simulink model "Drone_Flight_Model_StandAlone_KF_Steady"  (R2016b)
settings: Solver=FixedStepDiscrete  StartTime=0.0  StopTime=20  FixedStep=1/400  RelTol=1e-3  EnableMultiTasking=on
model workspace: external: MAT-File C:\Users\Patrick\Documents\TU\Integration project\AR_Drone_Models\Flight_Models\PD\parameters.mat (data not in the file)
undefined symbols (not defined in the file): accelerometerXyzGains, accelerometerXyzOffsets, Ak, Bk, botCamData, Ck, D_height, D_pitch, D_roll, D_yaw, DiscIntNeverNeededParam, Dk, Drone_StateModeType, dronePowerScaling, g, gyroXyzOffsets, I_height, M, magnetoXyzOffsets, Mass, P_height, P_pitch, P_roll, P_yaw, propDistance, yawTorqueC
libraries: simulink x17, dspstat3 x3, AR_Drone_Sensors x3, AR_Drone_Actuators x3, dspnetwork x2, visionanalysis x2, vrlib x2, AR_Drone_Video x1, AR_Drone_Positioning x1
(part 1 of 2)
settings Model: DataDictionary=ArDroneDataDictionary.sldd  ExtModeTrigDuration=48000  ExtModeLogAll=off  Creator=nraman  LastModifiedBy=s136161
settings ConfigSet: Description=This configuration set can be used to generate code that runs on the Parrot AR Drone 2.0 in Normal mode.
settings SolverCC: PositivePriorityOrder=on
settings DataIOCC: LimitDataPoints=on  SaveFormat=Array
settings OptimizationCC: DefaultParameterBehavior=Inlined  InlineInvariantSignals=on  LifeSpan=1  MaxStackSize=64
settings DebuggingCC: UnderspecifiedInitializationDetection=Classic  MergeDetectMultiDrivingBlocksExec=none  SFUnexpectedBacktrackingDiag=warning  SFNoUnconditionalDefaultTransitionDiag=warning
settings HardwareCC: ProdBitPerPointer=32  ProdBitPerSizeT=32  ProdBitPerPtrDiffT=32  ProdLargestAtomicInteger=Long  ProdLargestAtomicFloat=Double  ProdIntDivRoundTo=Undefined  ProdWordSize=32  ProdHWDeviceType=ARM Compatible->ARM Cortex
settings ModelReferenceCC: PropagateSignalLabelsOutOfModel=off
settings SFSimCC: SimUserSources=ArClock.c
settings SFSimCC: SimCustomHeaderCode=|
  | #include "IMU_Navdata.h"
  | #include "ArClock.h"
settings RTWCC: SystemTargetFile=ert.tlc  HardwareBoard=AR Drone 2 - Thread Timer Scheduler  TLCOptions=-aInlineSetEventsForThisBaseRateFcn=TLC_FALSE -aSuppressMultiTaskScheduler=TLC_FALSE -aRateBasedStepFcn=0  TemplateMakefile=ert_default_tmf  Description=Embedded Coder  RTWUseSimCustomCode=on  CustomSource=ArClock.c  Toolchain=Code Sourcery  BuildConfiguration=Faster Runs
settings RTWCC: CustomHeaderCode=|
  | #include "IMU_Navdata.h"
  | #include "ArClock.h"
settings CodeAppCC: IgnoreCustomStorageClasses=off
settings ERTTargetCC: SupportComplex=off  SupportVariableSizeSignals=on  ExtModeMexArgs='192.168.1.1' 1 17725  SuppressUnreachableDefaultCases=off
settings ConfigComp: CovMetricSettings=dw  CovHtmlReporting=on  CovSaveCumulativeToWorkspaceVar=on  CovSaveSingleToWorkspaceVar=on  CovExternalEMLEnable=off

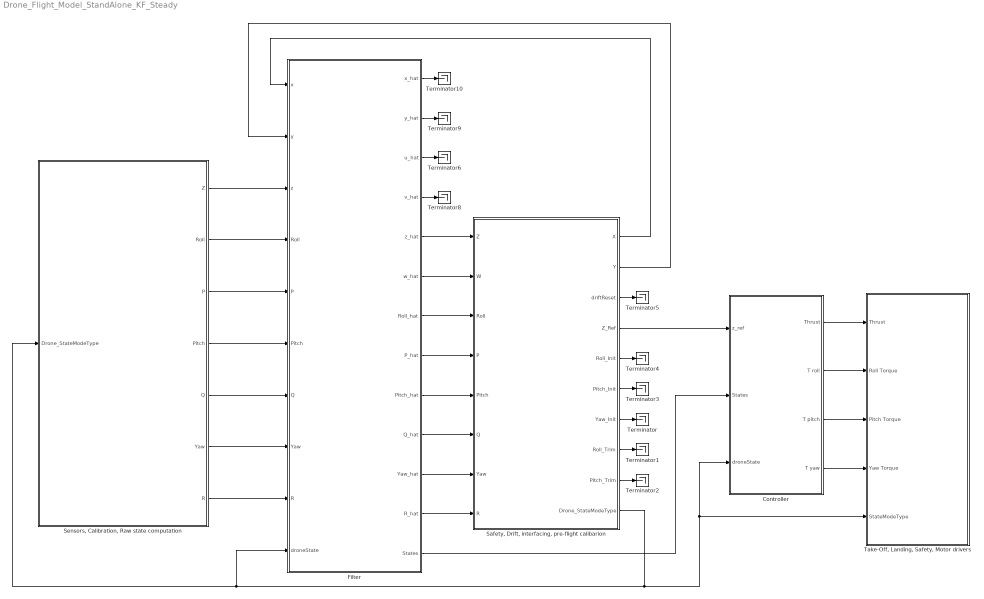
== system Drone_Flight_Model_StandAlone_KF_Steady ==
  Controller : Subsystem
  Filter : Subsystem
  "Safety, Drift, interfacing, pre-flight calibarion" : Subsystem
      settings: OpenFcn=msgbox('Please do not alter the functionality in the pre-made blocks.','Warning');
  "Sensors, Calibration, Raw state computation" : Subsystem
      settings: OpenFcn=msgbox('Please do not alter the functionality in the pre-made blocks.','Warning');
  "Take-Off, Landing, Safety, Motor drivers" : Subsystem
      settings: OpenFcn=msgbox('Please do not alter the functionality in the pre-made blocks.','Warning');
  Terminator{,1..6,8..10} (10 alike) : Terminator
  wires:
  "Safety, Drift, interfacing, pre-flight calibarion"/10(Drone_StateModeType) -> Filter/10(droneState), "Sensors, Calibration, Raw state computation"/1(Drone_StateModeType), Controller/3(droneState), "Take-Off, Landing, Safety, Motor drivers"/5(StateModeType)
  "Sensors, Calibration, Raw state computation"/1(Z) -> Filter/3(z)
  Filter/12(R_hat) -> "Safety, Drift, interfacing, pre-flight calibarion"/8(R)
  Filter/11(Yaw_hat) -> "Safety, Drift, interfacing, pre-flight calibarion"/7(Yaw)
  Filter/10(Q_hat) -> "Safety, Drift, interfacing, pre-flight calibarion"/6(Q)
  Filter/9(Pitch_hat) -> "Safety, Drift, interfacing, pre-flight calibarion"/5(Pitch)
  Filter/8(P_hat) -> "Safety, Drift, interfacing, pre-flight calibarion"/4(P)
  Filter/7(Roll_hat) -> "Safety, Drift, interfacing, pre-flight calibarion"/3(Roll)
  "Sensors, Calibration, Raw state computation"/2(Roll) -> Filter/4(Roll)
  "Sensors, Calibration, Raw state computation"/4(Pitch) -> Filter/6(Pitch)
  "Sensors, Calibration, Raw state computation"/3(P) -> Filter/5(P)
  "Sensors, Calibration, Raw state computation"/5(Q) -> Filter/7(Q)
  "Sensors, Calibration, Raw state computation"/6(Yaw) -> Filter/8(Yaw)
  "Sensors, Calibration, Raw state computation"/7(R) -> Filter/9(R)
  Filter/5(z_hat) -> "Safety, Drift, interfacing, pre-flight calibarion"/1(Z)
  "Safety, Drift, interfacing, pre-flight calibarion"/1(X) -> Filter/1(x)
  "Safety, Drift, interfacing, pre-flight calibarion"/2(Y) -> Filter/2(y)
  "Safety, Drift, interfacing, pre-flight calibarion"/9(Pitch_Trim) -> Terminator2/1
  "Safety, Drift, interfacing, pre-flight calibarion"/8(Roll_Trim) -> Terminator1/1
  "Safety, Drift, interfacing, pre-flight calibarion"/7(Yaw_Init) -> Terminator/1
  "Safety, Drift, interfacing, pre-flight calibarion"/6(Pitch_Init) -> Terminator3/1
  "Safety, Drift, interfacing, pre-flight calibarion"/5(Roll_Init) -> Terminator4/1
  "Safety, Drift, interfacing, pre-flight calibarion"/3(driftReset) -> Terminator5/1
  Filter/6(w_hat) -> "Safety, Drift, interfacing, pre-flight calibarion"/2(W)
  "Safety, Drift, interfacing, pre-flight calibarion"/4(Z_Ref) -> Controller/1(z_ref)
  Filter/13(States) -> Controller/2(States)
  Controller/1(Thrust) -> "Take-Off, Landing, Safety, Motor drivers"/1(Thrust)
  Controller/2(T roll) -> "Take-Off, Landing, Safety, Motor drivers"/2(Roll Torque)
  Controller/3(T pitch) -> "Take-Off, Landing, Safety, Motor drivers"/3(Pitch Torque)
  Controller/4(T yaw) -> "Take-Off, Landing, Safety, Motor drivers"/4(Yaw Torque)
  Filter/1(x_hat) -> Terminator10/1
  Filter/2(y_hat) -> Terminator9/1
  Filter/3(u_hat) -> Terminator6/1
  Filter/4(v_hat) -> Terminator8/1

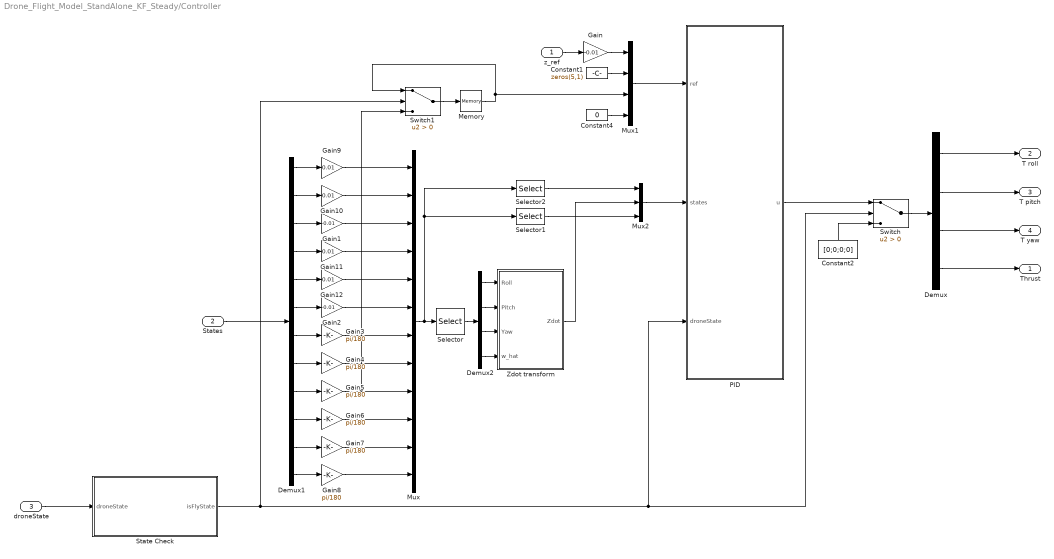
== system Drone_Flight_Model_StandAlone_KF_Steady/Controller ==
  z_ref : Inport
  States : Inport  Port=2
  droneState : Inport  Port=3
  Constant1 : Constant  Value=zeros(5,1)
  Constant2 : Constant  Value=[0;0;0;0]
  Constant4 : Constant  Value=0
  Demux : Demux
  Demux1 : Demux  Outputs=12
  Demux2 : Demux
  Gain : Gain  Gain=-0.01
  Gain1 : Gain  Gain=-0.01
  Gain{9..12} (4 alike) : Gain  Gain=0.01
  Gain2 : Gain  Gain=-0.01
  Gain{3..8} (6 alike) : Gain  Gain=pi/180
  Memory : Memory
  Mux : Mux  Inputs=12
  Mux1 : Mux
  Mux2 : Mux  Inputs=3
  PID : Subsystem
  Selector : Selector  InputPortWidth=12  IndexOptions=Index vector (dialog)  Indices=[7 8 9 6]  OutputSizes=1
  Selector1 : Selector  InputPortWidth=12  IndexOptions=Index vector (dialog)  Indices=[7 10 8 11 9 12]  OutputSizes=1
  Selector2 : Selector  InputPortWidth=12  IndexOptions=Index vector (dialog)  Indices=[3]  OutputSizes=1
  State Check : Subsystem
  Switch : Switch  Criteria=u2 > Threshold  InputSameDT=on
  Switch1 : Switch  Criteria=u2 > Threshold
  Zdot transform : Subsystem
  Thrust : Outport
  T roll : Outport  Port=2
  T pitch : Outport  Port=3
  T yaw : Outport  Port=4
  wires:
  Switch/1 -> Demux/1
  Constant2/1 -> Switch/3
  droneState/1 -> State Check/1(droneState)
  Demux1/7 -> Gain3/1
  Demux1/6 -> Gain2/1
  Demux1/3 -> Gain1/1
  z_ref/1 -> Gain/1
  Mux1/1 -> PID/1(ref)
  Gain/1 -> Mux1/1
  Gain1/1 -> Mux/3
  Gain2/1 -> Mux/6
  Gain3/1 -> Mux/7
  Gain4/1 -> Mux/8
  Gain5/1 -> Switch1/3, Mux/9
  Gain6/1 -> Mux/10
  Gain8/1 -> Mux/12
  Demux1/5 -> Gain12/1
  Gain12/1 -> Mux/5
  Demux1/4 -> Gain11/1
  Demux1/2 -> Gain10/1
  Gain10/1 -> Mux/2
  Gain11/1 -> Mux/4
  Gain9/1 -> Mux/1
  Demux1/1 -> Gain9/1
  PID/1(u) -> Switch/1
  State Check/1(isFlyState) -> Switch1/2, Switch/2, PID/3(droneState)
  Gain7/1 -> Mux/11
  Switch1/1 -> Memory/1
  Demux/2 -> T pitch/1
  Demux/1 -> T roll/1
  Demux/3 -> T yaw/1
  Demux1/9 -> Gain5/1
  Demux1/8 -> Gain4/1
  Demux1/10 -> Gain6/1
  Demux1/11 -> Gain7/1
  Demux1/12 -> Gain8/1
  Demux/4 -> Thrust/1
  States/1 -> Demux1/1
  Mux/1 -> Selector2/1, Selector1/1, Selector/1
  Selector/1 -> Demux2/1
  Demux2/1 -> Zdot transform/1(Roll)
  Demux2/2 -> Zdot transform/2(Pitch)
  Demux2/3 -> Zdot transform/3(Yaw)
  Demux2/4 -> Zdot transform/4(w_hat)
  Mux2/1 -> PID/2(states)
  Zdot transform/1(Zdot) -> Mux2/2
  Selector1/1 -> Mux2/3
  Selector2/1 -> Mux2/1
  Constant1/1 -> Mux1/2
  Constant4/1 -> Mux1/4
  Memory/1 -> Mux1/3, Switch1/1

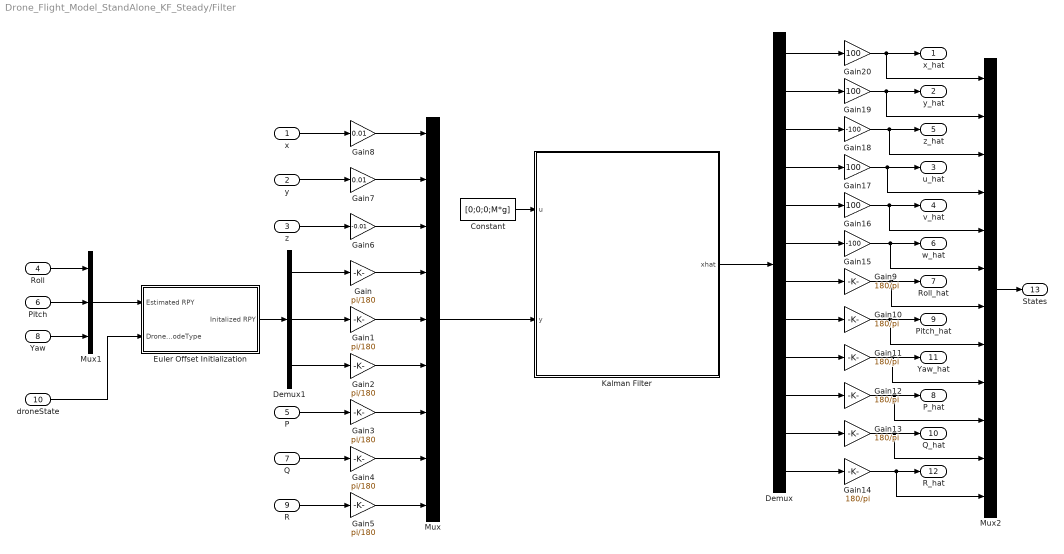
== system Drone_Flight_Model_StandAlone_KF_Steady/Filter ==
  x : Inport
  y : Inport  Port=2
  z : Inport  Port=3
  Roll : Inport  Port=4
  P : Inport  Port=5
  Pitch : Inport  Port=6
  Q : Inport  Port=7
  Yaw : Inport  Port=8
  R : Inport  Port=9
  droneState : Inport  Port=10
  Constant : Constant  Value=[0;0;0;M*g]
  Demux : Demux  Outputs=12
  Demux1 : Demux  Outputs=3
  Euler Offset Initialization : Subsystem
  Gain{,1..5} (6 alike) : Gain  Gain=pi/180
  Gain{9..14} (6 alike) : Gain  Gain=180/pi
  Gain15 : Gain  Gain=-100
  Gain{16..17,19..20} (4 alike) : Gain  Gain=100
  Gain18 : Gain  Gain=-100
  Gain6 : Gain  Gain=-0.01
  Gain7 : Gain  Gain=0.01
  Gain8 : Gain  Gain=0.01
  Kalman Filter : Subsystem
  Mux : Mux  Inputs=9
  Mux1 : Mux  Inputs=3
  Mux2 : Mux  Inputs=12
  x_hat : Outport
  y_hat : Outport  Port=2
  u_hat : Outport  Port=3
  v_hat : Outport  Port=4
  z_hat : Outport  Port=5
  w_hat : Outport  Port=6
  Roll_hat : Outport  Port=7
  P_hat : Outport  Port=8
  Pitch_hat : Outport  Port=9
  Q_hat : Outport  Port=10
  Yaw_hat : Outport  Port=11
  R_hat : Outport  Port=12
  States : Outport  Port=13
  wires:
  x/1 -> Gain8/1
  R/1 -> Gain5/1
  Q/1 -> Gain4/1
  P/1 -> Gain3/1
  Demux1/3 -> Gain2/1
  Demux1/2 -> Gain1/1
  Demux1/1 -> Gain/1
  z/1 -> Gain6/1
  y/1 -> Gain7/1
  Gain/1 -> Mux/4
  Gain1/1 -> Mux/5
  Gain2/1 -> Mux/6
  Gain3/1 -> Mux/7
  Gain4/1 -> Mux/8
  Gain5/1 -> Mux/9
  Gain7/1 -> Mux/2
  Gain8/1 -> Mux/1
  Demux/2 -> Gain19/1
  Demux/4 -> Gain17/1
  Demux/5 -> Gain16/1
  Demux/6 -> Gain15/1
  Demux/7 -> Gain9/1
  Demux/8 -> Gain10/1
  Demux/9 -> Gain11/1
  Demux/11 -> Gain13/1
  Demux/12 -> Gain14/1
  Gain9/1 -> Mux2/7, Roll_hat/1
  Gain10/1 -> Mux2/8, Pitch_hat/1
  Gain11/1 -> Mux2/9, Yaw_hat/1
  Gain12/1 -> Mux2/10, P_hat/1
  Gain13/1 -> Mux2/11, Q_hat/1
  Gain14/1 -> Mux2/12, R_hat/1
  Gain15/1 -> Mux2/6, w_hat/1
  Gain16/1 -> Mux2/5, v_hat/1
  Gain17/1 -> Mux2/4, u_hat/1
  Gain18/1 -> Mux2/3, z_hat/1
  Gain19/1 -> Mux2/2, y_hat/1
  Gain20/1 -> Mux2/1, x_hat/1
  Gain6/1 -> Mux/3
  Demux/1 -> Gain20/1
  Demux/10 -> Gain12/1
  Demux/3 -> Gain18/1
  Kalman Filter/1(xhat) -> Demux/1
  droneState/1 -> Euler Offset Initialization/2(Drone_StateModeType)
  Mux1/1 -> Euler Offset Initialization/1(Estimated RPY)
  Yaw/1 -> Mux1/3
  Pitch/1 -> Mux1/2
  Roll/1 -> Mux1/1
  Euler Offset Initialization/1(Initalized RPY) -> Demux1/1
  Mux2/1 -> States/1
  Constant/1 -> Kalman Filter/1(u)
  Mux/1 -> Kalman Filter/2(y)

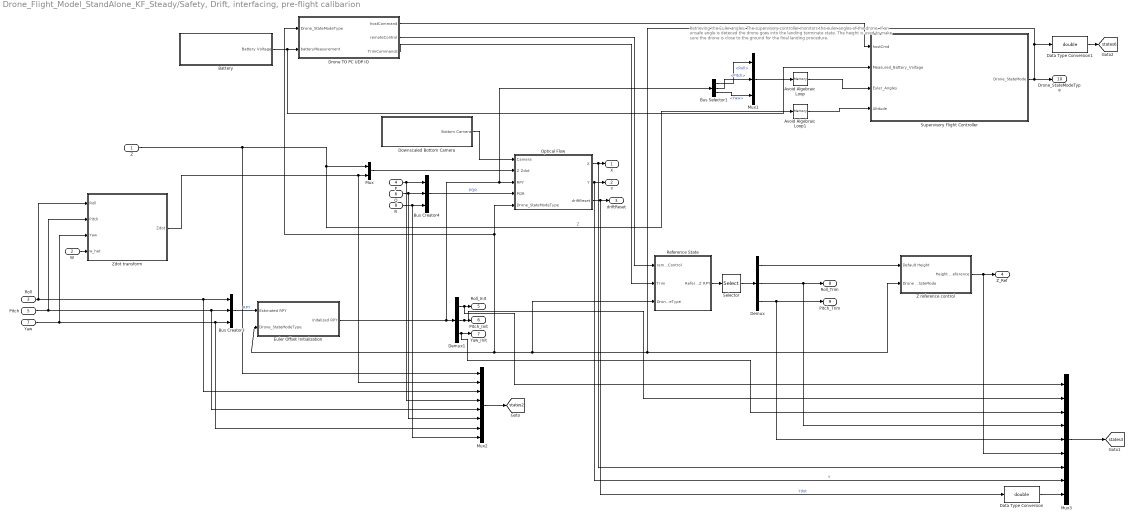
== system Drone_Flight_Model_StandAlone_KF_Steady/Safety, Drift, interfacing, pre-flight calibarion ==
  note: Retrieving the Euler angles:
      | The supervisory controller monitors the euler angles of the drone.
      | If an unsafe angle is deteced the drone goes into the landing terminate state.
      | The height is used to make sure the drone is close to the ground for the final landing procedure.
  Z : Inport
  W : Inport  Port=2
  Roll : Inport  Port=3
  P : Inport  Port=4
  Pitch : Inport  Port=5
  Q : Inport  Port=6
  Yaw : Inport  Port=7
  R : Inport  Port=8
  Avoid Algebraic Loop : Memory  InheritSampleTime=on
  Avoid Algebraic Loop1 : Memory  InheritSampleTime=on
  "Battery " : Subsystem
  Bus Creator3 : BusCreator  Inputs=3
  Bus Creator4 : BusCreator  Inputs=3
  Bus Selector1 : BusSelector  OutputSignals=Roll,Pitch,Yaw
  Data Type Conversion : DataTypeConversion  OutDataTypeStr=double
  Data Type Conversion1 : DataTypeConversion  OutDataTypeStr=double
  Demux : Demux  Outputs=3
  Demux1 : Demux  Outputs=3
  Downscaled Bottom Camera : Subsystem
  Drone TO PC UDP IO : Subsystem
  Euler Offset Initialization : Subsystem
  Mux : Mux  Inputs=2
  Mux1 : Mux  Inputs=3
  Mux2 : Mux  Inputs=8
  Mux3 : Mux  Inputs=9
  Optical Flow : Subsystem
  Reference State : Subsystem
  Selector : Selector  InputPortWidth=6  IndexOptions=Index vector (dialog)  Indices=[3 4 5]  OutputSizes=1
  Supervisory Flight Controller : Stateflow chart  TreatAsAtomicUnit=on
  Z reference control : Subsystem
  Zdot transform : Subsystem
  X : Outport
  Y : Outport  Port=2
  driftReset : Outport  Port=3
  Z_Ref : Outport  Port=4
  Roll_Init : Outport  Port=5
  Pitch_Init : Outport  Port=6
  Yaw_Init : Outport  Port=7
  Roll_Trim : Outport  Port=8
  Pitch_Trim : Outport  Port=9
  Drone_StateModeType : Outport  Port=10
  tag scope: states2=global, states3=global, states6=global
  wires:
  Supervisory Flight Controller/1(" Drone_StateMode") -> Drone_StateModeType/1, Reference State/3(Drone_StateModeType), Euler Offset Initialization/2(Drone_StateModeType), Optical Flow/5(Drone_StateModeType), Drone TO PC UDP IO/1(Drone_StateModeType), Z reference control/2(Drone StateMode), Data Type Conversion1/1
  R/1 -> Mux2/8, Bus Creator4/3
  Mux1/1 -> Avoid Algebraic Loop/1
  Demux/1 -> Z reference control/1(Default Height)
  Bus Selector1/2 -> Mux1/2  "<Pitch>"
  Bus Selector1/1 -> Mux1/1  "<Roll>"
  Bus Selector1/3 -> Mux1/3  "<Yaw>"
  Z reference control/1(Height Reference) -> Mux3/6, Z_Ref/1
  Avoid Algebraic Loop/1 -> Supervisory Flight Controller/3(Euler_Angles)
  Euler Offset Initialization/1(Initalized RPY) -> Bus Selector1/1, Optical Flow/3(RPY), Demux1/1
  Pitch/1 -> Zdot transform/2(Pitch), Mux2/5, Bus Creator3/2
  Drone TO PC UDP IO/2(remoteControl) -> Reference State/1(remoteControl)
  Roll/1 -> Zdot transform/1(Roll), Mux2/3, Bus Creator3/1
  Bus Creator3/1 -> Euler Offset Initialization/1(Estimated RPY)  "RPY"
  "Battery "/1(Battery Voltage) -> Supervisory Flight Controller/2(Measured_Battery_Voltage), Drone TO PC UDP IO/2(batteryMeasurement)
  Downscaled Bottom Camera/1(Bottom Camera) -> Optical Flow/1(Camera)
  Drone TO PC UDP IO/1(hostCommand) -> Supervisory Flight Controller/1(hostCmd)
  Bus Creator4/1 -> Optical Flow/4(PQR)  "PQR"
  Zdot transform/1(Zdot) -> Mux2/2, Mux/2
  Mux/1 -> Optical Flow/2(Z Zdot)
  P/1 -> Mux2/4, Bus Creator4/1
  Avoid Algebraic Loop1/1 -> Supervisory Flight Controller/4(Altitude)
  Drone TO PC UDP IO/3(TrimCommands) -> Reference State/2(Trim)
  Z/1 -> Mux2/1, Mux/1, Avoid Algebraic Loop1/1  "Z"
  Q/1 -> Mux2/6, Bus Creator4/2
  Demux/3 -> Mux3/5, Pitch_Trim/1
  Demux/2 -> Mux3/4, Roll_Trim/1
  Demux1/1 -> Mux3/1, Roll_Init/1
  Demux1/2 -> Mux3/2, Pitch_Init/1
  Demux1/3 -> Mux3/3, Yaw_Init/1
  Mux2/1 -> [states2]
  Mux3/1 -> [states3]
  Optical Flow/1(X) -> Mux3/7, X/1
  Optical Flow/2(Y) -> Mux3/8, Y/1  "Y"
  Optical Flow/3(driftReset) -> Data Type Conversion/1, driftReset/1  "Ydot"
  Selector/1 -> Demux/1
  Reference State/1(Reference XYZ RPY) -> Selector/1
  Data Type Conversion/1 -> Mux3/9
  Data Type Conversion1/1 -> [states6]
  Yaw/1 -> Zdot transform/3(Yaw), Mux2/7, Bus Creator3/3
  W/1 -> Zdot transform/4(w_hat)

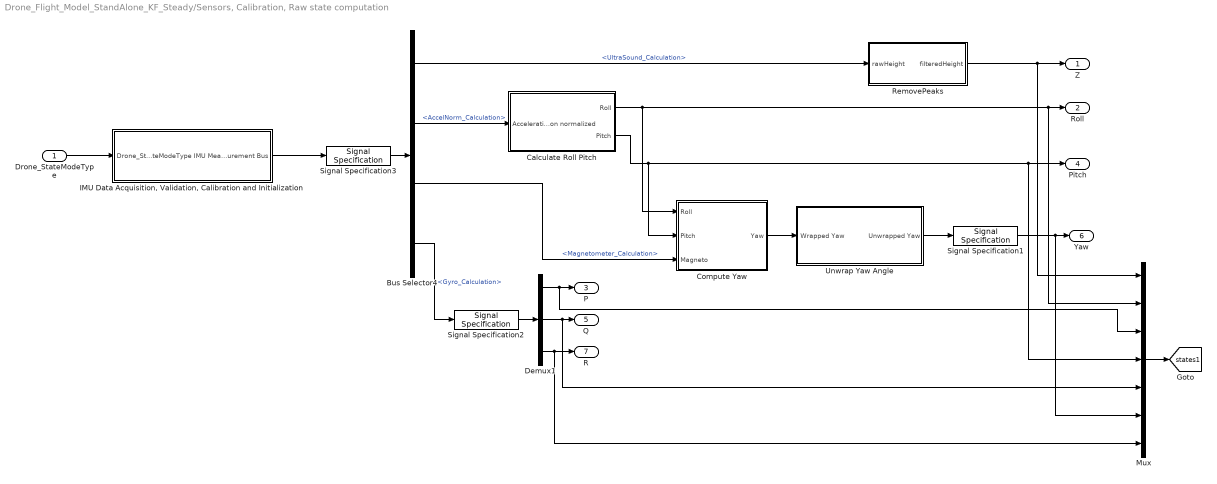
== system Drone_Flight_Model_StandAlone_KF_Steady/Sensors, Calibration, Raw state computation ==
  Drone_StateModeType : Inport
  Bus Selector4 : BusSelector  OutputSignals=UltraSound_Calculation,AccelNorm_Calculation,Magnetometer_Calculation,Gyro_Calculation
  Calculate Roll Pitch : Subsystem
  Compute Yaw : MATLAB Function  TreatAsAtomicUnit=on
  Demux1 : Demux  Outputs=3
  "IMU Data Acquisition, Validation, Calibration and Initialization" : Subsystem
  Mux : Mux  Inputs=7
  RemovePeaks : MATLAB Function  TreatAsAtomicUnit=on  mask{peakThreshold=40, peakHeightCounterThreshold=400}
      mask prompts: peakThreshold "Maxmimum height difference [cm]"; peakHeightCounterThreshold "How long a peak should be ignored [ticks]"
  Signal Specification1 : SignalSpecification  SampleTime=1/400
  Signal Specification2 : SignalSpecification  SampleTime=1/400
  Signal Specification3 : SignalSpecification  SampleTime=1/400
  Unwrap Yaw Angle : Subsystem
  Z : Outport
  Roll : Outport  Port=2
  P : Outport  Port=3
  Pitch : Outport  Port=4
  Q : Outport  Port=5
  Yaw : Outport  Port=6
  R : Outport  Port=7
  tag scope: states1=global
  wires:
  Signal Specification2/1 -> Demux1/1
  Bus Selector4/4 -> Signal Specification2/1  "<Gyro_Calculation>"
  Drone_StateModeType/1 -> "IMU Data Acquisition, Validation, Calibration and Initialization"/1(Drone_StateModeType)
  Demux1/2 -> Mux/5, Q/1
  Demux1/1 -> Mux/3, P/1
  Compute Yaw/1(Yaw) -> Unwrap Yaw Angle/1(Wrapped Yaw)
  Bus Selector4/2 -> Calculate Roll Pitch/1(Acceleration normalized)  "<AccelNorm_Calculation>"
  "IMU Data Acquisition, Validation, Calibration and Initialization"/1(IMU Measurement Bus) -> Signal Specification3/1
  Bus Selector4/1 -> RemovePeaks/1(rawHeight)  "<UltraSound_Calculation>"
  Bus Selector4/3 -> Compute Yaw/3(Magneto)  "<Magnetometer_Calculation>"
  Calculate Roll Pitch/2(Pitch) -> Mux/4, Pitch/1, Compute Yaw/2(Pitch)
  Calculate Roll Pitch/1(Roll) -> Mux/2, Roll/1, Compute Yaw/1(Roll)
  Unwrap Yaw Angle/1(Unwrapped Yaw) -> Signal Specification1/1
  Demux1/3 -> Mux/7, R/1
  Signal Specification1/1 -> Mux/6, Yaw/1
  RemovePeaks/1(filteredHeight) -> Mux/1, Z/1
  Signal Specification3/1 -> Bus Selector4/1
  Mux/1 -> [states1]

== system Drone_Flight_Model_StandAlone_KF_Steady/Take-Off, Landing, Safety, Motor drivers ==
  Thrust : Inport
  Roll Torque : Inport  Port=2
  Pitch Torque : Inport  Port=3
  Yaw Torque : Inport  Port=4
  StateModeType : Inport  Port=5
  AR Drone Motors : Subsystem
  Landing/TakeOff Sequence Controller : Subsystem
  Motor Cutoff/Initialize Controller : Subsystem
  Mux : Mux
  Scale to indivdual motors : Gain  Gain=0.25
  tag scope: states4=global
  wires:
  Landing/TakeOff Sequence Controller/3(Pitch Control) -> AR Drone Motors/3(Pitch Command)
  Landing/TakeOff Sequence Controller/4(Yaw Control) -> AR Drone Motors/4(Yaw Command)
  Landing/TakeOff Sequence Controller/1(Attitude Control) -> AR Drone Motors/1(Attitude Command)
  Landing/TakeOff Sequence Controller/2(Roll Control) -> AR Drone Motors/2(Roll Command)
  StateModeType/1 -> Landing/TakeOff Sequence Controller/2(Drone StateModeType), Motor Cutoff/Initialize Controller/2(Drone StateModeType)
  Thrust/1 -> Mux/1
  Yaw Torque/1 -> Mux/4
  Pitch Torque/1 -> Mux/3
  Roll Torque/1 -> Mux/2
  Motor Cutoff/Initialize Controller/1(Controls) -> Landing/TakeOff Sequence Controller/1(Controls)
  Mux/1 -> Scale to indivdual motors/1, [states4]
  Scale to indivdual motors/1 -> Motor Cutoff/Initialize Controller/1(Hover Controls)

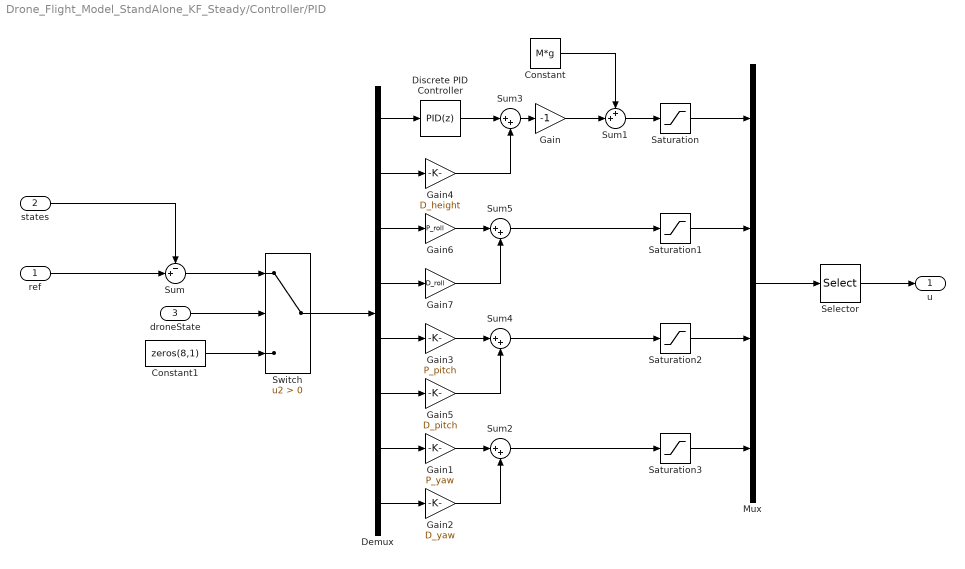
== system Drone_Flight_Model_StandAlone_KF_Steady/Controller/PID ==
  ref : Inport
  states : Inport  Port=2
  droneState : Inport  Port=3
  Constant : Constant  Value=M*g
  Constant1 : Constant  Value=zeros(8,1)
  Demux : Demux  Outputs=8
  Discrete PID Controller : simulink/Continuous/PID Controller  Controller=PID  TimeDomain=Discrete-time  SampleTime=-1  IntegratorMethod=Forward Euler  FilterMethod=Forward Euler  Form=Parallel  UseFilter=off  ControllerParametersSource=internal  P=P_height  I=I_height  D=0  N=100  InitialConditionSource=internal  InitialConditionForIntegrator=0  InitialConditionForFilter=0  ExternalReset=none  LimitOutput=off  UpperSaturationLimit=inf  LowerSaturationLimit=-inf  LinearizeAsGain=off  AntiWindupMode=none  Kb=1  TrackingMode=off  Kt=1  PParamMin=[]  PParamMax=[]  IParamMin=[]  IParamMax=[]  DParamMin=[]  DParamMax=[]  NParamMin=[]  NParamMax=[]  KbParamMin=[]  KbParamMax=[]  KtParamMin=[]  KtParamMax=[]  POutMin=[]  POutMax=[]  IOutMin=[]  IOutMax=[]  DOutMin=[]  DOutMax=[]  NOutMin=[]  NOutMax=[]  KbOutMin=[]  KbOutMax=[]  KtOutMin=[]  KtOutMax=[]  IntegratorOutMin=[]  IntegratorOutMax=[]  FilterOutMin=[]  FilterOutMax=[]  SumOutMin=[]  SumOutMax=[]  SumI1OutMin=[]  SumI1OutMax=[]  SumI2OutMin=[]  SumI2OutMax=[]  SumI3OutMin=[]  SumI3OutMax=[]  SumDOutMin=[]  SumDOutMax=[]  SaturationOutMin=[]  SaturationOutMax=[]  IntegratorContinuousStateAttributes=''  IntegratorStateMustResolveToSignalObject=off  IntegratorRTWStateStorageClass=Auto  FilterContinuousStateAttributes=''  FilterStateMustResolveToSignalObject=off  FilterRTWStateStorageClass=Auto  DifferentiatorICPrevScaledInput=0  DifferentiatorOutMin=[]  DifferentiatorOutMax=[]
  Gain : Gain  Gain=-1
  Gain1 : Gain  Gain=P_yaw
  Gain2 : Gain  Gain=D_yaw
  Gain3 : Gain  Gain=P_pitch
  Gain4 : Gain  Gain=D_height
  Gain5 : Gain  Gain=D_pitch
  Gain6 : Gain  Gain=P_roll
  Gain7 : Gain  Gain=D_roll
  Mux : Mux
  Saturation : Saturate  UpperLimit=8  LowerLimit=0
  Saturation1 : Saturate  UpperLimit=0.2  LowerLimit=-0.2
  Saturation2 : Saturate  UpperLimit=0.2  LowerLimit=-0.2
  Saturation3 : Saturate  UpperLimit=0.4  LowerLimit=-0.4
  Selector : Selector  InputPortWidth=4  IndexOptions=Index vector (dialog)  Indices=[2 3 4 1]  OutputSizes=1
  Sum : Sum  Inputs=-+|
  Sum1 : Sum  Inputs=++|
  Sum{2..5} (4 alike) : Sum  Inputs=|++
  Switch : Switch  Criteria=u2 > Threshold  InputSameDT=on
  u : Outport
  wires:
  Mux/1 -> Selector/1
  Gain/1 -> Sum1/2
  Constant/1 -> Sum1/1
  Sum1/1 -> Saturation/1
  Sum/1 -> Switch/1
  Switch/1 -> Demux/1
  droneState/1 -> Switch/2
  ref/1 -> Sum/2
  states/1 -> Sum/1
  Constant1/1 -> Switch/3
  Gain2/1 -> Sum2/2
  Gain1/1 -> Sum2/1
  Demux/7 -> Gain1/1
  Demux/8 -> Gain2/1
  Demux/2 -> Gain4/1
  Gain4/1 -> Sum3/2
  Sum3/1 -> Gain/1
  Discrete PID Controller/1 -> Sum3/1
  Demux/1 -> Discrete PID Controller/1
  Sum5/1 -> Saturation1/1
  Saturation1/1 -> Mux/2
  Saturation/1 -> Mux/1
  Saturation2/1 -> Mux/3
  Sum2/1 -> Saturation3/1
  Selector/1 -> u/1
  Saturation3/1 -> Mux/4
  Gain5/1 -> Sum4/2
  Gain3/1 -> Sum4/1
  Sum4/1 -> Saturation2/1
  Demux/6 -> Gain5/1
  Demux/5 -> Gain3/1
  Gain7/1 -> Sum5/2
  Gain6/1 -> Sum5/1
  Demux/4 -> Gain7/1
  Demux/3 -> Gain6/1

== system Drone_Flight_Model_StandAlone_KF_Steady/Controller/State Check ==
  droneState : Inport
  Logical Operator : Logic  Operator=OR  AllPortsSameDT=off  OutDataTypeStr=boolean
  compare1 : RelationalOperator  Operator===  OutDataTypeStr=boolean  RndMeth=Nearest
  compare2 : RelationalOperator  Operator===  OutDataTypeStr=boolean  RndMeth=Nearest
  ref state1 : simulink/Sources/Enumerated Constant  OutDataTypeStr=Enum: Drone_StateModeType  Value=Drone_StateModeType.Drift_Compensated_Flight  SampleTime=inf
  ref state2 : simulink/Sources/Enumerated Constant  OutDataTypeStr=Enum: Drone_StateModeType  Value=Drone_StateModeType.Landing_Descent  SampleTime=inf
  isFlyState : Outport
  wires:
  Logical Operator/1 -> isFlyState/1
  compare2/1 -> Logical Operator/2
  ref state2/1 -> compare2/2
  ref state1/1 -> compare1/1
  compare1/1 -> Logical Operator/1
  droneState/1 -> compare2/1, compare1/2

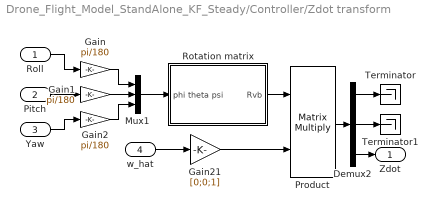
== system Drone_Flight_Model_StandAlone_KF_Steady/Controller/Zdot transform ==
  Roll : Inport
  Pitch : Inport  Port=2
  Yaw : Inport  Port=3
  w_hat : Inport  Port=4
  Demux2 : Demux  Outputs=3
  Gain : Gain  Gain=pi/180
  Gain1 : Gain  Gain=pi/180
  Gain2 : Gain  Gain=pi/180
  Gain21 : Gain  Gain=[0;0;1]
  Mux1 : Mux  Inputs=3
  Product : Product  Multiplication=Matrix(*)
  Rotation matrix : Subsystem
  Terminator : Terminator
  Terminator1 : Terminator
  Zdot : Outport
  wires:
  Product/1 -> Demux2/1
  Rotation matrix/1(Rvb) -> Product/1
  Gain21/1 -> Product/2
  Mux1/1 -> Rotation matrix/1(phi theta psi)
  w_hat/1 -> Gain21/1
  Yaw/1 -> Gain2/1
  Demux2/3 -> Zdot/1
  Pitch/1 -> Gain1/1
  Roll/1 -> Gain/1
  Gain/1 -> Mux1/1
  Gain1/1 -> Mux1/2
  Gain2/1 -> Mux1/3
  Demux2/1 -> Terminator/1
  Demux2/2 -> Terminator1/1

== system Drone_Flight_Model_StandAlone_KF_Steady/Filter/Euler Offset Initialization ==
  Estimated RPY : Inport
  Drone_StateModeType : Inport  Port=2
  Add : Sum  Inputs=+-  OutDataTypeStr=Inherit: Same as first input
  Bus Creator4 : BusCreator  Inputs=3
  Compute RPY Offset : dspstat3/Mean  run=on  reset_popup=Rising edge  directionMode=Each column  dimension=1  roiEnable=off  roiType=Rectangles  roiPortion=Entire ROI  roiOutput=Individual statistics for each ROI  roiFlag=off  outputDataTypeStr=Inherit: Same as accumulator  outputLastDataTypeStr=Inherit: Same as accumulator  outputMin=[]  outputMax=[]  roundingMode=Floor  overflowMode=off
  Demux : Demux  Outputs=3
  Enumerated Constant2 : simulink/Sources/Enumerated Constant  OutDataTypeStr=Enum: Drone_StateModeType  Value=Drone_StateModeType.Initialize_Computation  SampleTime=inf
      settings: AttributesFormatString=%<Value>
  Offset Calc Reset Boolean : RelationalOperator  Operator===  OutDataTypeStr=boolean  RndMeth=Nearest
  Offset Memory : Memory  X0=[0 0 0]  InheritSampleTime=on
  Output Selector : Switch  Criteria=u2 > Threshold  InputSameDT=on
  Output Selector Reset Boolean : RelationalOperator  Operator=~=  OutDataTypeStr=boolean  RndMeth=Nearest
  Signal Specification : SignalSpecification  Dimensions=3
  Initalized RPY : Outport
  wires:
  Offset Calc Reset Boolean/1 -> Compute RPY Offset/2
  Estimated RPY/1 -> Add/1, Compute RPY Offset/1
  Output Selector Reset Boolean/1 -> Output Selector/2
  Compute RPY Offset/1 -> Output Selector/3
  Output Selector/1 -> Add/2, Offset Memory/1
  Add/1 -> Signal Specification/1
  Drone_StateModeType/1 -> Output Selector Reset Boolean/2, Offset Calc Reset Boolean/2
  Offset Memory/1 -> Output Selector/1
  Enumerated Constant2/1 -> Output Selector Reset Boolean/1, Offset Calc Reset Boolean/1
  Demux/1 -> Bus Creator4/1  "Roll"
  Demux/2 -> Bus Creator4/2  "Pitch"
  Demux/3 -> Bus Creator4/3  "Yaw"
  Bus Creator4/1 -> Initalized RPY/1  "RPY"
  Signal Specification/1 -> Demux/1

== system Drone_Flight_Model_StandAlone_KF_Steady/Filter/Kalman Filter ==
  u : Inport
  y : Inport  Port=2
  Constant : Constant
  Discrete State-Space : DiscreteStateSpace  A=Ak  B=Bk  C=Ck  D=Dk  SampleTime=-1
  Mux : Mux  Inputs=2
  Mux1 : Mux  Inputs=2
  xhat : Outport
  wires:
  Mux/1 -> Discrete State-Space/1
  y/1 -> Mux/2
  Discrete State-Space/1 -> xhat/1
  u/1 -> Mux1/1
  Constant/1 -> Mux1/2
  Mux1/1 -> Mux/1

== system Drone_Flight_Model_StandAlone_KF_Steady/Safety, Drift, interfacing, pre-flight calibarion/Battery  ==
  note: Battery Measurement:
      | The battery driver measures in deciVolts. After converting to Volts the signal is smoothed,
      | this is needed because the voltage briefly drops below operating conditions during take-off.
  Battery Voltage Measurement : AR_Drone_Sensors/Battery Voltage Measurement  SFunctionSpec=void BatteryMeasure_step(single y1[1])  SampleTime=1/400
  Data Type Conversion : DataTypeConversion  OutDataTypeStr=double
  Smooth Battery Voltage : DiscreteTransferFcn  Numerator=[0.05]  Denominator=[1 -0.95]
  dV to V : Gain  Gain=0.1
  Battery Voltage : Outport
  wires:
  Battery Voltage Measurement/1 -> Data Type Conversion/1
  dV to V/1 -> Smooth Battery Voltage/1
  Smooth Battery Voltage/1 -> Battery Voltage/1
  Data Type Conversion/1 -> dV to V/1

== system Drone_Flight_Model_StandAlone_KF_Steady/Safety, Drift, interfacing, pre-flight calibarion/Downscaled Bottom Camera ==
  note: Downscaled bottom camera:
      | The bottom camera can be sampled at up to 30 fps and has a resolution of 320x240.
      | Processing the full image is too computationally intensive so the image is down sampled.
  AR_Drone_Bottom_Camera : AR_Drone_Video/AR_Drone_Bottom_Camera  SFunctionSpec=videoGrabImage2(uint8 y1[153600])  SampleTime=botCamData.sampleTime  ShowSpec=off
  Downscale Chroma Image : MATLAB Function  TreatAsAtomicUnit=on  mask{width=botCamData.resolution(1), height=botCamData.resolution(2), downScaleFactor=botCamData.downScaleFactor}
      mask prompts: downScaleFactor "down scale factor"
  Bottom Camera : Outport
  wires:
  AR_Drone_Bottom_Camera/1 -> Downscale Chroma Image/1(YCbCr422In)
  Downscale Chroma Image/1(cameraChroma) -> Bottom Camera/1

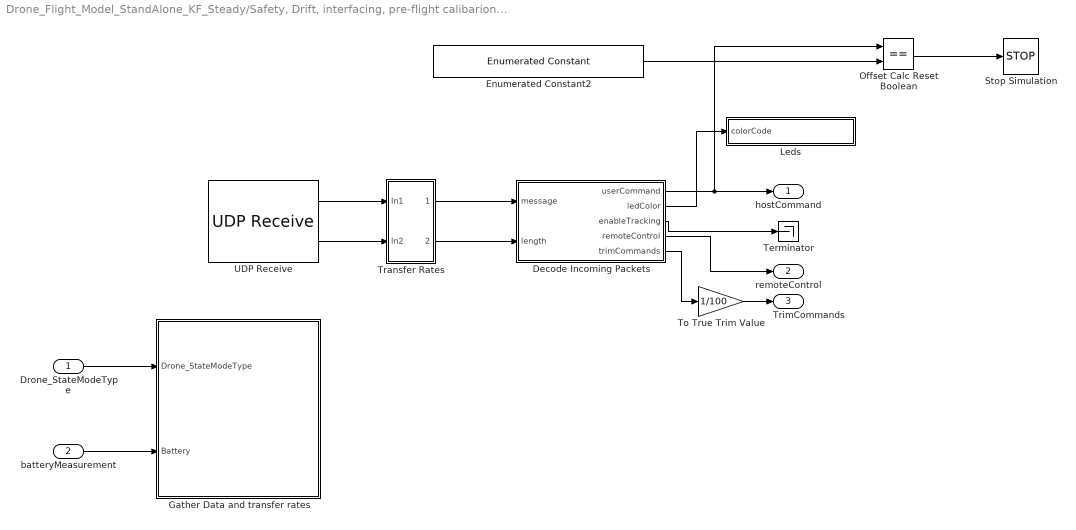
== system Drone_Flight_Model_StandAlone_KF_Steady/Safety, Drift, interfacing, pre-flight calibarion/Drone TO PC UDP IO ==
  Drone_StateModeType : Inport
  batteryMeasurement : Inport  Port=2
  Decode Incoming Packets : MATLAB Function  TreatAsAtomicUnit=on  mask{maxUpdateDelay=1600}
      mask prompts: maxUpdateDelay "Maxmimum update delay"
  Enumerated Constant2 : simulink/Sources/Enumerated Constant  OutDataTypeStr=Enum: Drone_StateModeType  Value=Drone_StateModeType.Landing_Terminate  SampleTime=inf
      settings: AttributesFormatString=%<Value>
  Gather Data and transfer rates : Subsystem  mask{udpSampleTime=4/400}
      mask prompts: udpSampleTime "UDP Sample Time"
  Leds : Subsystem
  Offset Calc Reset Boolean : RelationalOperator  Operator===  OutDataTypeStr=boolean  RndMeth=Nearest
  Stop Simulation : Stop
  Terminator : Terminator
  To True Trim Value : Gain  Gain=1/100  OutDataTypeStr=double
  Transfer Rates : Subsystem
  UDP Receive : dspnetwork/UDP Receive  localURL='0.0.0.0'  localPort=24000  remoteURL='192.168.1.2'  remotePort=-1  recvBufferSize=2048  dims=6  signalDatatype=uint8  isVarSize=off  showBlockingTime=off  blockingTime=0  sampletime=4/400
  hostCommand : Outport
  remoteControl : Outport  Port=2
  TrimCommands : Outport  Port=3
  wires:
  Decode Incoming Packets/1(userCommand) -> hostCommand/1, Offset Calc Reset Boolean/1
  UDP Receive/1 -> Transfer Rates/1(In1)
  UDP Receive/2 -> Transfer Rates/2(In2)
  Transfer Rates/1(Out1) -> Decode Incoming Packets/1(message)
  Transfer Rates/2(Out2) -> Decode Incoming Packets/2(length)
  Decode Incoming Packets/2(ledColor) -> Leds/1(colorCode)
  Drone_StateModeType/1 -> Gather Data and transfer rates/1(Drone_StateModeType)
  batteryMeasurement/1 -> Gather Data and transfer rates/2(Battery)
  Decode Incoming Packets/3(enableTracking) -> Terminator/1
  Decode Incoming Packets/4(remoteControl) -> remoteControl/1
  Decode Incoming Packets/5(trimCommands) -> To True Trim Value/1
  To True Trim Value/1 -> TrimCommands/1
  Enumerated Constant2/1 -> Offset Calc Reset Boolean/2
  Offset Calc Reset Boolean/1 -> Stop Simulation/1

== system Drone_Flight_Model_StandAlone_KF_Steady/Safety, Drift, interfacing, pre-flight calibarion/Euler Offset Initialization ==
  note: Euler Offset Initialization
      | The Euler angles are calibrated each time before flight takes place during the
      | Drone_StateModeType.Initialize state. After calibration the Roll, Pitch and Yaw
      | of the drone before take off are assumed to be zero.
  Estimated RPY : Inport
  Drone_StateModeType : Inport  Port=2
  Add : Sum  Inputs=+-  OutDataTypeStr=Inherit: Same as first input
  Bus Creator4 : BusCreator  Inputs=3
  Compute RPY Offset : dspstat3/Mean  run=on  reset_popup=Rising edge  directionMode=Each column  dimension=1  roiEnable=off  roiType=Rectangles  roiPortion=Entire ROI  roiOutput=Individual statistics for each ROI  roiFlag=off  outputDataTypeStr=Inherit: Same as accumulator  outputLastDataTypeStr=Inherit: Same as accumulator  outputMin=[]  outputMax=[]  roundingMode=Floor  overflowMode=off
  Demux : Demux  Outputs=3
  Enumerated Constant2 : simulink/Sources/Enumerated Constant  OutDataTypeStr=Enum: Drone_StateModeType  Value=Drone_StateModeType.Initialize_Computation  SampleTime=inf
      settings: AttributesFormatString=%<Value>
  Offset Calc Reset Boolean : RelationalOperator  Operator===  OutDataTypeStr=boolean  RndMeth=Nearest
  Offset Memory : Memory  X0=[0 0 0]  InheritSampleTime=on
  Output Selector : Switch  Criteria=u2 > Threshold  InputSameDT=on
  Output Selector Reset Boolean : RelationalOperator  Operator=~=  OutDataTypeStr=boolean  RndMeth=Nearest
  Signal Specification : SignalSpecification  Dimensions=3
  Initalized RPY : Outport
  wires:
  Offset Calc Reset Boolean/1 -> Compute RPY Offset/2
  Estimated RPY/1 -> Add/1, Compute RPY Offset/1
  Output Selector Reset Boolean/1 -> Output Selector/2
  Compute RPY Offset/1 -> Output Selector/3
  Output Selector/1 -> Add/2, Offset Memory/1
  Add/1 -> Signal Specification/1
  Drone_StateModeType/1 -> Output Selector Reset Boolean/2, Offset Calc Reset Boolean/2
  Offset Memory/1 -> Output Selector/1
  Enumerated Constant2/1 -> Output Selector Reset Boolean/1, Offset Calc Reset Boolean/1
  Demux/1 -> Bus Creator4/1  "Roll"
  Demux/2 -> Bus Creator4/2  "Pitch"
  Demux/3 -> Bus Creator4/3  "Yaw"
  Bus Creator4/1 -> Initalized RPY/1  "RPY"
  Signal Specification/1 -> Demux/1

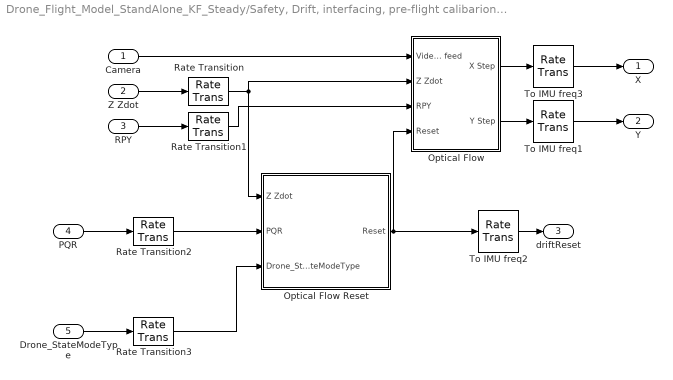
== system Drone_Flight_Model_StandAlone_KF_Steady/Safety, Drift, interfacing, pre-flight calibarion/Optical Flow ==
  Camera : Inport
  Z Zdot : Inport  Port=2
  RPY : Inport  Port=3
  PQR : Inport  Port=4
  Drone_StateModeType : Inport  Port=5
  Optical Flow : Subsystem
  Optical Flow Reset : Subsystem
  Rate Transition{,1..3} (4 alike) : RateTransition  OutPortSampleTime=botCamData.sampleTime
  To IMU freq1 : RateTransition  OutPortSampleTime=1/400
  To IMU freq2 : RateTransition  OutPortSampleTime=1/400
  To IMU freq3 : RateTransition  OutPortSampleTime=1/400
  X : Outport
  Y : Outport  Port=2
  driftReset : Outport  Port=3
  wires:
  Camera/1 -> Optical Flow/1(Video feed)
  Rate Transition/1 -> Optical Flow/2(Z Zdot), Optical Flow Reset/1(Z Zdot)
  Rate Transition1/1 -> Optical Flow/3(RPY)
  Optical Flow Reset/1(Reset) -> Optical Flow/4(Reset), To IMU freq2/1
  Z Zdot/1 -> Rate Transition/1
  RPY/1 -> Rate Transition1/1
  PQR/1 -> Rate Transition2/1
  Rate Transition2/1 -> Optical Flow Reset/2(PQR)
  Drone_StateModeType/1 -> Rate Transition3/1
  Rate Transition3/1 -> Optical Flow Reset/3(Drone_StateModeType)
  To IMU freq2/1 -> driftReset/1
  Optical Flow/1(X Step) -> To IMU freq3/1
  To IMU freq3/1 -> X/1
  Optical Flow/2(Y Step) -> To IMU freq1/1
  To IMU freq1/1 -> Y/1

== system Drone_Flight_Model_StandAlone_KF_Steady/Safety, Drift, interfacing, pre-flight calibarion/Reference State ==
  note: Setting the drone reference state:
      | The constant blocks in here can be changed to your desired reference state.
      | It is not recommended to set non zero reference states for anything other than the height and yaw.
      | The X and Y references are placeholders and have no effect.
  remoteControl : Inport
  Trim : Inport  Port=2
  Drone_StateModeType : Inport  Port=3
  Data Type Conversion : DataTypeConversion  OutDataTypeStr=double
  Default Height : Constant  Value=0.8
  MATLAB Function : MATLAB Function  TreatAsAtomicUnit=on
  Mux : Mux  Inputs=6
  Signal Specification : SignalSpecification  SampleTime=1/400
  Smooth Remote Input : DiscreteTransferFcn  Numerator=[0.25]  Denominator=[1 -0.75]
  To cm : Gain  Gain=100
  Reference XYZ RPY : Outport
  wires:
  Signal Specification/1 -> Reference XYZ RPY/1
  Mux/1 -> Smooth Remote Input/1
  remoteControl/1 -> Data Type Conversion/1
  Default Height/1 -> To cm/1
  To cm/1 -> MATLAB Function/1(defaultHeight)
  MATLAB Function/4(roll) -> Mux/4
  MATLAB Function/5(pitch) -> Mux/5
  MATLAB Function/3(z) -> Mux/3
  MATLAB Function/6(yaw) -> Mux/6
  MATLAB Function/2(y) -> Mux/2
  MATLAB Function/1(x) -> Mux/1
  Data Type Conversion/1 -> MATLAB Function/2(remoteControl)
  Drone_StateModeType/1 -> MATLAB Function/4(drone_StateModeType)
  Smooth Remote Input/1 -> Signal Specification/1
  Trim/1 -> MATLAB Function/3(trimCommands)

== system Drone_Flight_Model_StandAlone_KF_Steady/Safety, Drift, interfacing, pre-flight calibarion/Z reference control ==
  Default Height : Inport
  Drone StateMode : Inport  Port=2
  Landing Descent Reference : Subsystem
  Height Reference : Outport
  wires:
  Default Height/1 -> Landing Descent Reference/2(Height Reference In)
  Drone StateMode/1 -> Landing Descent Reference/1(Drone_StateModeType)
  Landing Descent Reference/1(Height Reference) -> Height Reference/1

== system Drone_Flight_Model_StandAlone_KF_Steady/Safety, Drift, interfacing, pre-flight calibarion/Zdot transform ==
  Roll : Inport
  Pitch : Inport  Port=2
  Yaw : Inport  Port=3
  w_hat : Inport  Port=4
  Demux2 : Demux  Outputs=3
  Gain : Gain  Gain=pi/180
  Gain1 : Gain  Gain=pi/180
  Gain2 : Gain  Gain=pi/180
  Gain21 : Gain  Gain=[0;0;1]
  Mux1 : Mux  Inputs=3
  Product : Product  Multiplication=Matrix(*)
  Rotation matrix : Subsystem
  Terminator : Terminator
  Terminator1 : Terminator
  Zdot : Outport
  wires:
  Product/1 -> Demux2/1
  Rotation matrix/1(Rvb) -> Product/1
  Gain21/1 -> Product/2
  Mux1/1 -> Rotation matrix/1(phi theta psi)
  w_hat/1 -> Gain21/1
  Yaw/1 -> Gain2/1
  Demux2/3 -> Zdot/1
  Pitch/1 -> Gain1/1
  Roll/1 -> Gain/1
  Gain/1 -> Mux1/1
  Gain1/1 -> Mux1/2
  Gain2/1 -> Mux1/3
  Demux2/1 -> Terminator/1
  Demux2/2 -> Terminator1/1

== system Drone_Flight_Model_StandAlone_KF_Steady/Sensors, Calibration, Raw state computation/Calculate Roll Pitch ==
  note: http://www.digikey.com/en/articles/techzone/2011/may/using-an-accelerometer-for-inclination-sensing
  Acceleration normalized : Inport
  Gain4 : Gain  Gain=180/pi
  Gain5 : Gain  Gain=180/pi
  MATLAB Function : MATLAB Function  TreatAsAtomicUnit=on
  Roll : Outport
  Pitch : Outport  Port=2
  wires:
  MATLAB Function/1(Roll) -> Gain4/1  "Roll"
  MATLAB Function/2(Pitch) -> Gain5/1  "Pitch"
  Gain4/1 -> Roll/1
  Gain5/1 -> Pitch/1
  Acceleration normalized/1 -> MATLAB Function/1(Ax_Ay_Az)

== system Drone_Flight_Model_StandAlone_KF_Steady/Sensors, Calibration, Raw state computation/IMU Data Acquisition, Validation, Calibration and Initialization ==
  Drone_StateModeType : Inport
  Inertial Measurement : AR_Drone_Sensors/Inertial Measurement  Ts=1/400  enableIMUReset=1
  Measurement Verification and Calibration : Subsystem
  Mux : Mux  Inputs=2
  Sensor Initialization : Subsystem
  IMU Measurement Bus : Outport
  tag scope: flags=global
  wires:
  Measurement Verification and Calibration/1(IMU Measurement Bus) -> Sensor Initialization/1(Measurement_Calculation_Bus)
  Inertial Measurement/3 -> Mux/2, Measurement Verification and Calibration/3(IMU Reset Flag)
  Sensor Initialization/1(Initalized Measurement_Calculation_Bus) -> IMU Measurement Bus/1
  Inertial Measurement/1 -> Measurement Verification and Calibration/1(IMU Data Bus)
  Inertial Measurement/2 -> Mux/1, Measurement Verification and Calibration/2(CheckSum)
  Drone_StateModeType/1 -> Sensor Initialization/2(Drone_StateModeType)
  Mux/1 -> [flags]

== system Drone_Flight_Model_StandAlone_KF_Steady/Sensors, Calibration, Raw state computation/Unwrap Yaw Angle ==
  Wrapped Yaw : Inport
  MATLAB Function : MATLAB Function  TreatAsAtomicUnit=on
  Memory : Memory  InheritSampleTime=on
  Unwrapped Yaw : Outport
  wires:
  Wrapped Yaw/1 -> Memory/1, MATLAB Function/1(wrappedYaw)
  MATLAB Function/1(unwrappedYaw) -> Unwrapped Yaw/1
  Memory/1 -> MATLAB Function/2(previousYaw)

== system Drone_Flight_Model_StandAlone_KF_Steady/Take-Off, Landing, Safety, Motor drivers/AR Drone Motors ==
  Attitude Command : Inport
  Roll Command : Inport  Port=2
  Pitch Command : Inport  Port=3
  Yaw Command : Inport  Port=4
  Demux3 : Demux
  Initialize_Actuators : AR_Drone_Actuators/Initialize_Actuators  ShowSpec=on
  MotorMixing : Subsystem
  Motors : AR_Drone_Actuators/Motors
  Terminator : Terminator
  tag scope: states5=global
  wires:
  Pitch Command/1 -> MotorMixing/3(pitch_command)
  Demux3/3 -> Motors/3
  Roll Command/1 -> MotorMixing/2(roll_command)
  Demux3/2 -> Motors/2
  Demux3/4 -> Motors/4
  Motors/1 -> Terminator/1
  Demux3/1 -> Motors/1
  Yaw Command/1 -> MotorMixing/4(yaw_command)
  Attitude Command/1 -> MotorMixing/1(altitude_command)
  MotorMixing/1(MotorCommands) -> [states5], Demux3/1

== system Drone_Flight_Model_StandAlone_KF_Steady/Take-Off, Landing, Safety, Motor drivers/Landing//TakeOff Sequence Controller ==
  Controls : Inport
  Drone StateModeType : Inport  Port=2
  Demux : Demux
  Landing/TakeOff Altitude Control : Subsystem
  Attitude Control : Outport
  Roll Control : Outport  Port=2
  Pitch Control : Outport  Port=3
  Yaw Control : Outport  Port=4
  wires:
  Controls/1 -> Demux/1
  Demux/4 -> Yaw Control/1
  Demux/2 -> Roll Control/1
  Demux/3 -> Pitch Control/1
  Drone StateModeType/1 -> Landing/TakeOff Altitude Control/1(Drone StateModeType)
  Demux/1 -> Landing/TakeOff Altitude Control/2(Attitude Hover Control)
  Landing/TakeOff Altitude Control/1(Attitude Control) -> Attitude Control/1

== system Drone_Flight_Model_StandAlone_KF_Steady/Take-Off, Landing, Safety, Motor drivers/Motor Cutoff//Initialize Controller ==
  note: Motor cutoff control:
      | If the drone state is not landing or controlled flight,
      | all PWM signals are set to 0.
  Hover Controls : Inport
  Drone StateModeType : Inport  Port=2
  MATLAB Function : MATLAB Function  TreatAsAtomicUnit=on
  Controls : Outport
  wires:
  Drone StateModeType/1 -> MATLAB Function/2(droneState)
  Hover Controls/1 -> MATLAB Function/1(hoverControls)
  MATLAB Function/1(motorControls) -> Controls/1

== system Drone_Flight_Model_StandAlone_KF_Steady/Controller/Zdot transform/Rotation matrix ==
  phi theta psi : Inport
  Rotm in euler : MATLAB Function  TreatAsAtomicUnit=on
  Transpose : Math  Operator=transpose  SaturateOnIntegerOverflow=on
  Rvb : Outport
  wires:
  phi theta psi/1 -> Rotm in euler/1(alpha)
  Rotm in euler/1(Rbv) -> Transpose/1
  Transpose/1 -> Rvb/1

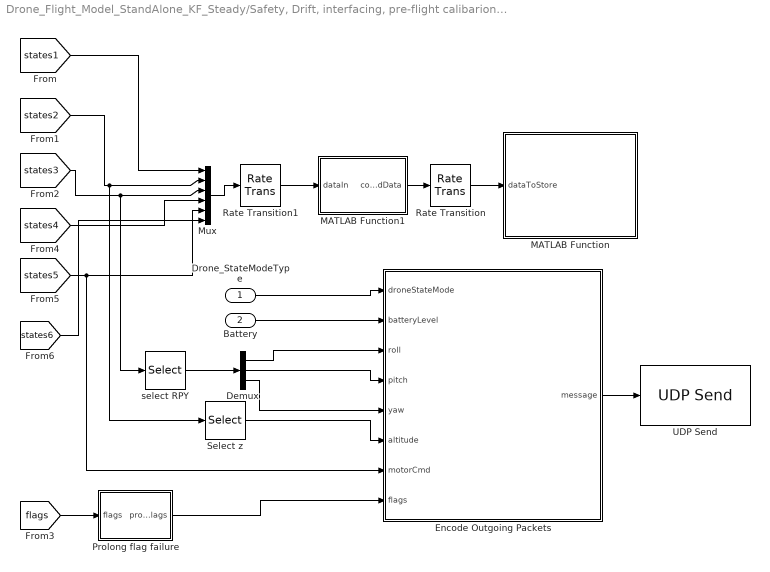
== system Drone_Flight_Model_StandAlone_KF_Steady/Safety, Drift, interfacing, pre-flight calibarion/Drone TO PC UDP IO/Gather Data and transfer rates ==
  Drone_StateModeType : Inport
  Battery : Inport  Port=2
  Demux : Demux  Outputs=3
  Encode Outgoing Packets : MATLAB Function  TreatAsAtomicUnit=on
  MATLAB Function : MATLAB Function  TreatAsAtomicUnit=on
  MATLAB Function1 : MATLAB Function  TreatAsAtomicUnit=on
  Mux : Mux  Inputs=6
  Prolong flag failure : MATLAB Function  TreatAsAtomicUnit=on
  Rate Transition : RateTransition  OutPortSampleTime=1/100
  Rate Transition1 : RateTransition  OutPortSampleTime=1/200
  Select z : Selector  InputPortWidth=8  IndexOptions=Index vector (dialog)  Indices=[1]  OutputSizes=1
  UDP Send : dspnetwork/UDP Send  remoteURL='192.168.1.2'  remotePort=23000  localURL='0.0.0.0'  localPortSource=Automatically determine  localPort=-1  sampletime=-1  blockPlatform=LINUX  separateLengthPort=0
  select RPY : Selector  InputPortWidth=9  IndexOptions=Index vector (dialog)  Indices=[1 2 3]  OutputSizes=1
  wires:
  [flags] -> Prolong flag failure/1(flags)
  [states1] -> Mux/1
  [states2] -> Select z/1, Mux/2
  [states3] -> select RPY/1, Mux/3
  [states4] -> Mux/4
  Mux/1 -> Rate Transition1/1
  Rate Transition/1 -> MATLAB Function/1(dataToStore)
  MATLAB Function1/1(combinedData) -> Rate Transition/1
  Rate Transition1/1 -> MATLAB Function1/1(dataIn)
  [states5] -> Mux/5, Encode Outgoing Packets/7(motorCmd)
  Encode Outgoing Packets/1(message) -> UDP Send/1
  select RPY/1 -> Demux/1
  Demux/1 -> Encode Outgoing Packets/3(roll)
  Demux/2 -> Encode Outgoing Packets/4(pitch)
  Demux/3 -> Encode Outgoing Packets/5(yaw)
  Prolong flag failure/1(prolongedFlags) -> Encode Outgoing Packets/8(flags)
  Battery/1 -> Encode Outgoing Packets/2(batteryLevel)
  Drone_StateModeType/1 -> Encode Outgoing Packets/1(droneStateMode)
  Select z/1 -> Encode Outgoing Packets/6(altitude)
  [states6] -> Mux/6

== system Drone_Flight_Model_StandAlone_KF_Steady/Safety, Drift, interfacing, pre-flight calibarion/Drone TO PC UDP IO/Leds ==
  colorCode : Inport
  LEDs : AR_Drone_Actuators/LEDs
  Rate Transition : RateTransition  OutPortSampleTime=1/20
  wires:
  Rate Transition/1 -> LEDs/3, LEDs/1, LEDs/2, LEDs/4
  colorCode/1 -> Rate Transition/1

== system Drone_Flight_Model_StandAlone_KF_Steady/Safety, Drift, interfacing, pre-flight calibarion/Drone TO PC UDP IO/Transfer Rates ==
  In1 : Inport
  In2 : Inport  Port=2
  Rate Transition1 : RateTransition  OutPortSampleTime=1/400
  Rate Transition2 : RateTransition  OutPortSampleTime=1/400
  Out1 : Outport
  Out2 : Outport  Port=2
  wires:
  In2/1 -> Rate Transition2/1
  Rate Transition2/1 -> Out2/1
  In1/1 -> Rate Transition1/1
  Rate Transition1/1 -> Out1/1

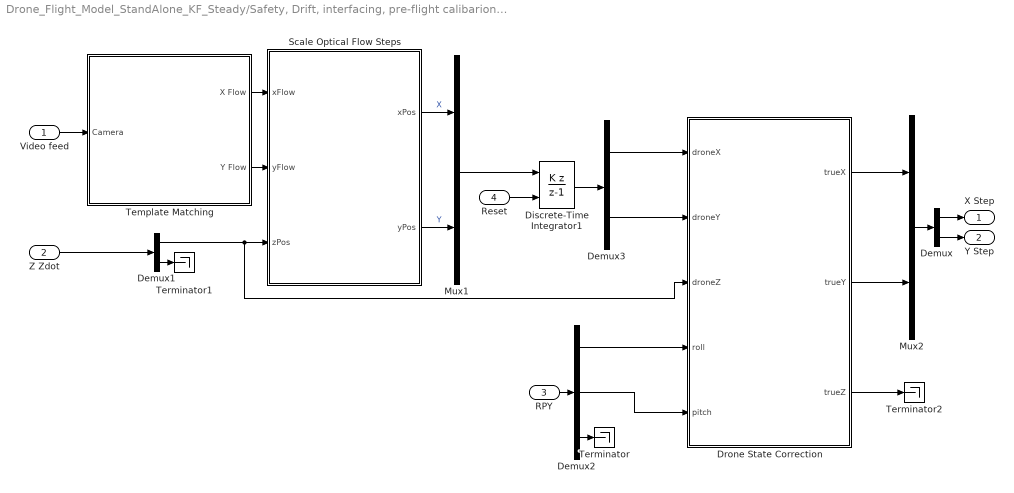
== system Drone_Flight_Model_StandAlone_KF_Steady/Safety, Drift, interfacing, pre-flight calibarion/Optical Flow/Optical Flow ==
  Video feed : Inport
  Z Zdot : Inport  Port=2
  RPY : Inport  Port=3
  Reset : Inport  Port=4
  Demux : Demux  Outputs=2
  Demux1 : Demux  Outputs=2
  Demux2 : Demux  Outputs=3
  Demux3 : Demux  Outputs=2
  Discrete-Time Integrator1 : DiscreteIntegrator  IntegratorMethod=Accumulation: Backward Euler  gainval=1  ExternalReset=level  InitialConditionSetting=State (most efficient)  SampleTime=-1  ICPrevOutput=DiscIntNeverNeededParam  ICPrevScaledInput=DiscIntNeverNeededParam
  Drone State Correction : MATLAB Function  TreatAsAtomicUnit=on
  Mux1 : Mux  Inputs=2
  Mux2 : Mux  Inputs=2
  Scale Optical Flow Steps : MATLAB Function  TreatAsAtomicUnit=on  mask{downScaleFactor=botCamData.downScaleFactor, FOV=botCamData.FOV}
      mask prompts: downScaleFactor "Camera Down Scale Factor"
  Template Matching : Subsystem
  Terminator : Terminator
  Terminator1 : Terminator
  Terminator2 : Terminator
  X Step : Outport
  Y Step : Outport  Port=2
  wires:
  Video feed/1 -> Template Matching/1(Camera)
  Template Matching/1(X Flow) -> Scale Optical Flow Steps/1(xFlow)
  Template Matching/2(Y Flow) -> Scale Optical Flow Steps/2(yFlow)
  Mux2/1 -> Demux/1
  Demux/1 -> X Step/1
  Demux/2 -> Y Step/1
  Demux1/1 -> Drone State Correction/3(droneZ), Scale Optical Flow Steps/3(zPos)
  Demux2/1 -> Drone State Correction/4(roll)
  Demux2/2 -> Drone State Correction/5(pitch)
  Z Zdot/1 -> Demux1/1
  RPY/1 -> Demux2/1
  Demux2/3 -> Terminator/1
  Demux1/2 -> Terminator1/1
  Drone State Correction/2(trueY) -> Mux2/2
  Drone State Correction/1(trueX) -> Mux2/1
  Drone State Correction/3(trueZ) -> Terminator2/1
  Scale Optical Flow Steps/1(xPos) -> Mux1/1  "X"
  Scale Optical Flow Steps/2(yPos) -> Mux1/2  "Y"
  Mux1/1 -> Discrete-Time Integrator1/1
  Reset/1 -> Discrete-Time Integrator1/2
  Discrete-Time Integrator1/1 -> Demux3/1
  Demux3/1 -> Drone State Correction/1(droneX)
  Demux3/2 -> Drone State Correction/2(droneY)

== system Drone_Flight_Model_StandAlone_KF_Steady/Safety, Drift, interfacing, pre-flight calibarion/Optical Flow/Optical Flow Reset ==
  Z Zdot : Inport
  PQR : Inport  Port=2
  Drone_StateModeType : Inport  Port=3
  Drone_StateMode Reset Condition : Subsystem
  Logical Operator : Logic  Operator=OR  Inputs=3  AllPortsSameDT=off  OutDataTypeStr=boolean
  PQR Reset Condition : Subsystem
  Zdot Reset condition : Subsystem
  Reset : Outport
  wires:
  Z Zdot/1 -> Zdot Reset condition/1(Z Zdot)
  PQR/1 -> PQR Reset Condition/1(PQR)
  Zdot Reset condition/1(Zdot Reset) -> Logical Operator/1
  Logical Operator/1 -> Reset/1
  PQR Reset Condition/1(PQR Reset) -> Logical Operator/2
  Drone_StateModeType/1 -> Drone_StateMode Reset Condition/1(Drone_StateMode)
  Drone_StateMode Reset Condition/1(Drone_StateMode Reset) -> Logical Operator/3

== system Drone_Flight_Model_StandAlone_KF_Steady/Safety, Drift, interfacing, pre-flight calibarion/Z reference control/Landing Descent Reference ==
  Drone_StateModeType : Inport
  Height Reference In : Inport  Port=2
  Descent Velocity [cm/s] : Constant  Value=20
  Enumerated Constant : simulink/Sources/Enumerated Constant  OutDataTypeStr=Enum: Drone_StateModeType  Value=Drone_StateModeType.Landing_Descent  SampleTime=inf
  Gain : Gain  Gain=1/400
  Landing Descent Boolean : RelationalOperator  Operator===  OutDataTypeStr=boolean  RndMeth=Nearest
  Memory : Memory
  Sum1 : Sum  Inputs=|+-
  Switch : Switch  Criteria=u2 > Threshold  InputSameDT=on
  Height Reference : Outport
  wires:
  Memory/1 -> Sum1/1
  Enumerated Constant/1 -> Landing Descent Boolean/2
  Switch/1 -> Height Reference/1, Memory/1
  Drone_StateModeType/1 -> Landing Descent Boolean/1
  Height Reference In/1 -> Switch/3
  Descent Velocity [cm/s]/1 -> Gain/1
  Landing Descent Boolean/1 -> Switch/2
  Sum1/1 -> Switch/1
  Gain/1 -> Sum1/2

== system Drone_Flight_Model_StandAlone_KF_Steady/Safety, Drift, interfacing, pre-flight calibarion/Zdot transform/Rotation matrix ==
  phi theta psi : Inport
  Rotm in euler : MATLAB Function  TreatAsAtomicUnit=on
  Transpose : Math  Operator=transpose  SaturateOnIntegerOverflow=on
  Rvb : Outport
  wires:
  phi theta psi/1 -> Rotm in euler/1(alpha)
  Rotm in euler/1(Rbv) -> Transpose/1
  Transpose/1 -> Rvb/1

== system Drone_Flight_Model_StandAlone_KF_Steady/Sensors, Calibration, Raw state computation/IMU Data Acquisition, Validation, Calibration and Initialization/Measurement Verification and Calibration ==
  IMU Data Bus : Inport  OutDataTypeStr=Bus: IMU_Packets
  CheckSum : Inport  Port=2
  IMU Reset Flag : Inport  Port=3
  Create Measurement Bus : AR_Drone_Positioning/Navigation System/Create Measurement Bus
  Measurement calibration correction : Subsystem
  Verify IMU Data : AR_Drone_Sensors/Verify IMU Data  discardPacketCount=25
  IMU Measurement Bus : Outport
  wires:
  CheckSum/1 -> Verify IMU Data/2
  IMU Reset Flag/1 -> Verify IMU Data/3
  Create Measurement Bus/1 -> Measurement calibration correction/1(MeasurementDataBus)
  IMU Data Bus/1 -> Verify IMU Data/1
  Verify IMU Data/1 -> Create Measurement Bus/1
  Measurement calibration correction/1(Measurement_Calculation_Bus) -> IMU Measurement Bus/1
